simulink model "FxLMS_wip"  (R2018b)
settings: Solver=FixedStepDiscrete  StartTime=0.0  StopTime=20  RelTol=1e-3  EnableMultiTasking=on
InitFcn:
  | % Sine wave generator to synthetically create the noise
  | A = [.01 .01 .02 .2 .3 .4 .3 .2 .1 .07 .02 .01]; La = length(A);
  | F0 = 60; k = 1:La; F = F0*k;
  | phase = rand(1,La); % Random initial phase
  | Fs = 44100;
  | SamplesPerFrame = 1;
  | 
  | % Initialize the coefficients for S(z)
  | 
  | % All frequency values are in Hz.
  | Fs = 44100;  % Sampling Frequency
  | 
  | N     = 16;    % Order
  | %Fpass = 300;  % Passband Frequency
  | %Fstop = 4000;  % Stopband Frequency
  | Fpass = 1000;  % Passband Frequency
  | Fstop = 3000;  % Stopband Frequency
  | Wpass = 1;     % Passband Weight
  | Wstop = 1;     % Stopband Weight
  | dens  = 20;    % Density Factor
  | 
  | % Calculate the coefficients using the FIRPM function.
  | b  = firpm(N, [0 Fpass Fstop Fs/2]/(Fs/2), [1 1 0 0], [Wpass Wstop], ...
  |            {dens});
  | 
  | SecondaryCoeffsEstimate = b;
undefined symbols (not defined in the file or in its folder): SecondaryPath
libraries: dspsrcs4 x2, dspsnks4 x1, dspadpt3 x1, dspindex x1
settings Model: Creator=The MathWorks, Inc.  LastModifiedBy=micha_000
settings DataIOCC: ExternalInput=[t,u]  SaveFormat=Array  SaveOutput=off  SaveTime=off
settings OptimizationCC: LifeSpan=inf  SimCompilerOptimization=on
settings DebuggingCC: AllowSymbolicDim=off  SFUnexpectedBacktrackingDiag=warning  SFNoUnconditionalDefaultTransitionDiag=warning  SFExecutionAtInitializationDiag=none
settings HardwareCC: ProdBitPerPointer=32  ProdBitPerSizeT=32  ProdBitPerPtrDiffT=32  ProdLargestAtomicFloat=None  ProdIntDivRoundTo=Undefined  ProdEndianess=Unspecified  ProdWordSize=32  ProdHWDeviceType=32-bit Generic
settings ModelReferenceCC: PropagateSignalLabelsOutOfModel=off
settings SFSimCC: SimUseLocalCustomCode=off
settings RTWCC: RTWUseLocalCustomCode=off
settings CodeAppCC: StateflowObjectComments=on
settings GRTTargetCC: TargetLangStandard=C89/C90 (ANSI)  GeneratePreprocessorConditionals=Disable all
settings ConfigComp: CovMetricSettings=dw  CovHtmlReporting=on  CovSaveCumulativeToWorkspaceVar=on  CovSaveSingleToWorkspaceVar=on  CovShowResultsExplorer=off  CovExternalEMLEnable=off

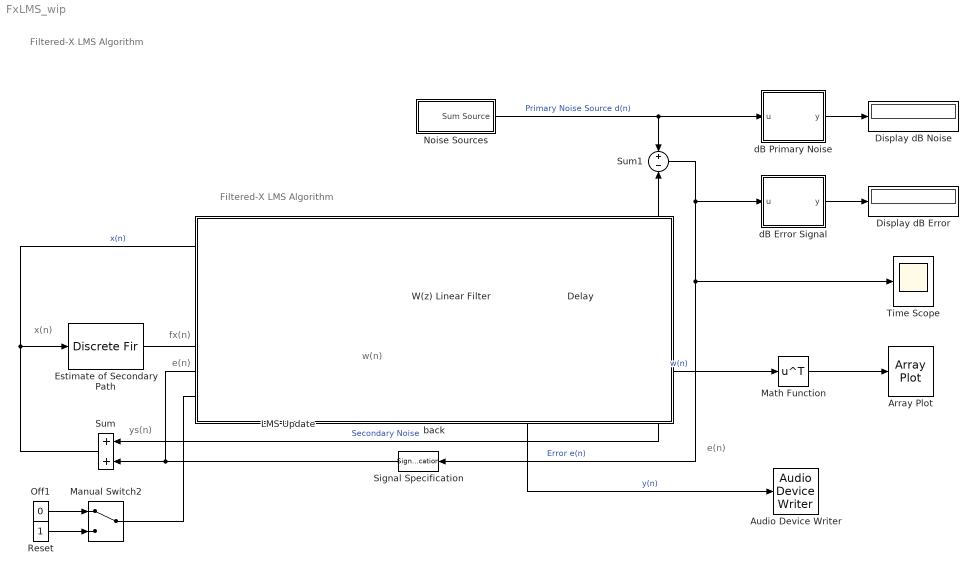
== system FxLMS_wip ==
  note: w(n)
  note: e(n)
  note: fx(n)
  note: Filtered-X LMS Algorithm
  note: e(n)
  note: Filtered-X LMS Algorithm
  note: x(n)
  note: ys(n)
  Array Plot : ArrayPlot
  Audio Device Writer : dspsnks4/Audio Device Writer  Driver=DirectSound  Device=Default  InheritSampleRate=on  SampleRate=44100  BitDepth=16-bit integer  BufferSize=4096  NumBuffers=10  DefaultOutputChannelMapping=on  OutputChannelMapping=1:2  OutputNumUnderrunSamples=off  DriverIdx=1  DeviceWarnFlag=''
  "Delay " : Subsystem
  Display dB Error : Display
  Display dB Noise : Display
  Estimate of Secondary Path : DiscreteFir  Coefficients=SecondaryCoeffsEstimate  InputProcessing=Columns as channels (frame based)  AccumDataTypeStr=Inherit: Same as product output  OutDataTypeStr=Inherit: Same as input
  LMS Update : dspadpt3/LMS Update  Method=LMS  Length=65  StepSizeSource=Property  StepSize=5e-4  LeakageFactor=1 -4*eps('single')  InitialConditions=0  EnableAdaptInput=off  EnableResetInput=on  SimulateUsing=Code generation
      settings: SourceProductName=DSP System Toolbox  SourceProductBaseCode=DS
  Manual Switch2 : ManualSwitch
  Math Function : Math  Operator=transpose  SaturateOnIntegerOverflow=on
  Noise Sources : Subsystem
  Off1 : Constant  Value=0  OutDataTypeStr=boolean
  Reset : Constant  OutDataTypeStr=boolean
  Signal Specification : SignalSpecification  Dimensions=[1 1]
  Sum : Sum
  Sum1 : Sum  Inputs=+-
  Time Scope : Scope
  W(z) Linear Filter : DiscreteFir  CoefSource=Input port  Coefficients=SecondaryPath  InputProcessing=Columns as channels (frame based)  AccumDataTypeStr=Inherit: Same as product output  OutDataTypeStr=Inherit: Same as input
      settings: InputPortMap=u0,u1
  back : Subsystem
  dB Error Signal : MATLAB Function  TreatAsAtomicUnit=on
  dB Primary Noise : MATLAB Function  TreatAsAtomicUnit=on
  wires:
  Estimate of Secondary Path/1 -> LMS Update/1
  Sum1/1 -> dB Error Signal/1(u), Time Scope/1, Signal Specification/1  "Error e(n)"
  Sum/1 -> Estimate of Secondary Path/1, W(z) Linear Filter/1  "x(n)"
  Noise Sources/1(Sum Source) -> dB Primary Noise/1(u), Sum1/1  "Primary Noise Source d(n)"
  dB Error Signal/1(y) -> Display dB Error/1
  dB Primary Noise/1(y) -> Display dB Noise/1
  LMS Update/1 -> W(z) Linear Filter/2, Math Function/1  "w(n)"
  Math Function/1 -> Array Plot/1
  "Delay "/1(ys(n)) -> Sum/1, Sum1/2  "Secondary Noise"
  W(z) Linear Filter/1 -> "Delay "/1(y(n)), Audio Device Writer/1  "y(n)"
  Signal Specification/1 -> LMS Update/2, Sum/2
  Off1/1 -> Manual Switch2/1
  Reset/1 -> Manual Switch2/2
  Manual Switch2/1 -> LMS Update/3

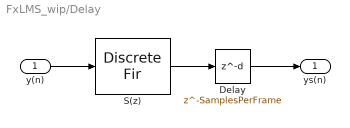
== system FxLMS_wip/Delay  ==
  y(n) : Inport
  Delay : Delay  DelayLength=SamplesPerFrame  InitialCondition=0  InputProcessing=Columns as channels (frame based)
  S(z) : DiscreteFir  Coefficients=SecondaryCoeffsEstimate  InputProcessing=Columns as channels (frame based)  AccumDataTypeStr=Inherit: Same as product output  OutDataTypeStr=Inherit: Same as input
  ys(n) : Outport
  wires:
  Delay/1 -> ys(n)/1
  S(z)/1 -> Delay/1
  y(n)/1 -> S(z)/1

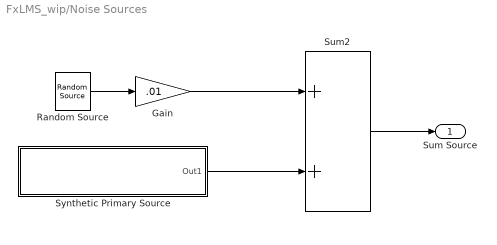
== system FxLMS_wip/Noise Sources ==
  Gain : Gain  Gain=.01
  Random Source : dspsrcs4/Random Source  SrcType=Gaussian  NormMethod=Ziggurat  CltLength=12  MinVal=0  MaxVal=1  MeanVal=0  VarVal=1  RepMode=Specify seed  rawSeed=1  IsInherit=off  SampMode=Discrete  SampTime=1/Fs  SampFrame=SamplesPerFrame  DataType=Double  OutComplex=Real  OutputFrames=off
  Sum2 : Sum
  "Synthetic Primary Source " : Subsystem
  Sum Source : Outport
  wires:
  Random Source/1 -> Gain/1
  "Synthetic Primary Source "/1(Out1) -> Sum2/2
  Gain/1 -> Sum2/1
  Sum2/1 -> Sum Source/1

== system FxLMS_wip/back ==

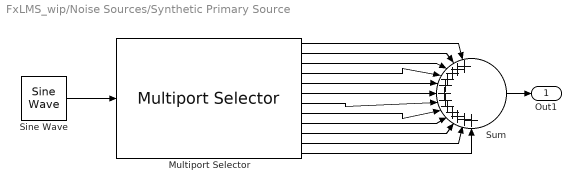
== system FxLMS_wip/Noise Sources/Synthetic Primary Source  ==
  Multiport Selector : dspindex/Multiport Selector  rowsOrCols=Columns  idxCellArray={ 1,2,3,4,5,6,7,8,9,10,11,12}  idxErrMode=Clip Index
  Sine Wave : dspsrcs4/Sine Wave  Amplitude=A  Frequency=F  Phase=phase  SampleMode=Discrete  OutComplex=Real  CompMethod=Trigonometric fcn  TableSize=Speed  SampleTime=1/Fs  SamplesPerFrame=SamplesPerFrame  ResetState=Restart at time zero  OutputFrames=on  dataType=double  wordLen=16  udDataType=sfix(16)  fracBitsMode=Best precision  numFracBits=15  OutDataTypeStr=double  LastOutDataTypeStr=double
  Sum : Sum  Inputs=|++++++++++++
  Out1 : Outport
  wires:
  Multiport Selector/9 -> Sum/9
  Multiport Selector/1 -> Sum/1
  Multiport Selector/11 -> Sum/11
  Multiport Selector/4 -> Sum/4
  Multiport Selector/6 -> Sum/6
  Multiport Selector/5 -> Sum/5
  Sine Wave/1 -> Multiport Selector/1
  Multiport Selector/2 -> Sum/2
  Multiport Selector/3 -> Sum/3
  Multiport Selector/10 -> Sum/10
  Multiport Selector/8 -> Sum/8
  Multiport Selector/7 -> Sum/7
  Sum/1 -> Out1/1
  Multiport Selector/12 -> Sum/12

== matlab function FxLMS_wip/dB Error Signal ==
  data: u input; y output
function y  = fcn(u)
%#codegen

persistent yLast

if(isempty(yLast))
    yLast = 0;
end

% 1st order smoothing filter
% a = Ts / (Tau + Ts)
% Let Tau = 0.5 seconds
a = (1/44100) / (0.5 + (1/44100));
y = (1-a)*yLast + a*10*log10(mean(u.^2));
yLast = y;

== matlab function FxLMS_wip/dB Primary Noise ==
  data: u input; y output
function y  = fcn(u)
%#codegen

persistent yLast

if(isempty(yLast))
    yLast = 0;
end

% 1st order smoothing filter
% a = Ts / (Tau + Ts)
% Let Tau = 0.5 seconds
a = (1/44100) / (0.5 + (1/44100));
y = (1-a)*yLast + a*10*log10(mean(u.^2));
yLast = y;
